simulink model "Final_Model_Building_2_AirflowAdded_BufferMode"  (R2022a)
settings: Solver=FixedStepAuto  StartTime=0.0  StopTime=24*3600  FixedStep=5  RelTol=1e-3
values from neighbouring files (symbols this model uses):
  Aux_Threshold = 52    [Setup_Code_EWASP_VC.m]
  buildingAge = 2005    [Setup_Code_EWASP_VC.m]
  ceilingHeight = 2.4    [Setup_Code_EWASP_VC.m]
  conductiveHconnectMatrix = [ ... (first row only)    [Setup_Code_EWASP_VC.m]
  cRoofGreen = 100000    [Setup_Code_EWASP_VC.m]
  Defrost_After_Time = 30    [Setup_Code_EWASP_VC.m]
  DHWDemandProfile = occFreegainHotwaterElecTestPassiveOcc3(:,3)    [Setup_Code_EWASP_VC.m]
  Elec_Max = Elec_Max*(30/24.2)    [Setup_Code_EWASP_VC.m]
  Elec_Mid = Elec_Mid*(30/24.2)    [Setup_Code_EWASP_VC.m]
  Elec_Min = Elec_Min*(30/24.2)    [Setup_Code_EWASP_VC.m]
  ElecDemandProfile = occFreegainHotwaterElecTestPassiveOcc3(:,4)    [Setup_Code_EWASP_VC.m]
  ElecFixed = [Elec_Max(6,2) Elec_Max(6,4) Elec_Max(6,6) Elec_Max(6,7) ... (first row only)    [Setup_Code_EWASP_VC.m]
  floorOrCeilingArea = floorOrCeilingArea*1.15    [Setup_Code_EWASP_VC.m]
  freegain = occFreegainHotwaterElecTestPassiveOcc3(:,2)-max(occupancy)*25    [Setup_Code_EWASP_VC.m]
  furnitureModelOn = 1    [Setup_Code_EWASP_VC.m]
  Heat_Max = Heat_Max*(30/24.2)    [Setup_Code_EWASP_VC.m]
  Heat_Mid = Heat_Mid*(30/24.2)    [Setup_Code_EWASP_VC.m]
  Heat_Min = Heat_Min*(30/24.2)    [Setup_Code_EWASP_VC.m]
  HeatFixed = [Heat_Max(6,2) Heat_Max(6,4) Heat_Max(6,6) Heat_Max(6,7) ... (first row only)    [Setup_Code_EWASP_VC.m]
  HeatingOnProfile = repmat(HeatingOnProfile,365,1)    [Setup_Code_EWASP_VC.m]
  HEX_ReturnLowerLimit = 52.5    [Setup_Code_EWASP_VC.m]
  HEX_ReturnUpperLimit = 55    [Setup_Code_EWASP_VC.m]
  LeakMultiplier = 1+(2*(rand()-0.5)/10)    [Setup_Code_EWASP_VC.m]
  maxOcc = max(occupancyProfile)    [Setup_Code_EWASP_VC.m]
  NESW_wallArea = max(NESW_Lengths*ceilingHeight-NESW_Windows,0)    [Setup_Code_EWASP_VC.m]
  NESW_Windows = [ ... (first row only)    [Setup_Code_EWASP_VC.m]
  numRooms = roomCount    [Setup_Code_EWASP_VC.m]
  occupancy = occupancyProfile    [Setup_Code_EWASP_VC.m]
  offsetDays = 0    [Setup_Code_EWASP_VC.m]
  overChargeSeries = repmat(overChargeSeries,365,1)    [Setup_Code_EWASP_VC.m]
  pumpChoice = pumpChoices(MinIndex,1)    [Setup_Code_EWASP_VC.m]
  pumpRamp = 180    [Setup_Code_EWASP_VC.m]
  RoofIrradiance = Flat_NS_EW_RoofIrradiance(:,1)    [Setup_Code_EWASP_VC.m]
  roofStartTemp = ones(11,1)*20    [Setup_Code_EWASP_VC.m]
  rooftype = 0    [Setup_Code_EWASP_VC.m]
  RoomDataMatrix = [zeros(1,12);ones(1,12)*wallDensity;zeros(1,12);ones(1,12)*wallU;ones(1,12)*windowU;ones(1,12)*floorU;ones(1,12)*ceilingU;zeros(1,12);windowArea, 0;floorOrCeilingArea;zeros(1,12);floorOrCeilingArea*ceilingHeight]    [Setup_Code_EWASP_VC.m]
  roomVol = roomVol*1.15    [Setup_Code_EWASP_VC.m]
  slabStartTemp = (GroundTempTimeSeries(offsetDays*1440+1,1)+thermostatSetting)/2    [Setup_Code_EWASP_VC.m]
  SlackRequest = zeros(1440,1)    [Setup_Code_EWASP_VC.m]
  SolarThermalExists = 0    [Setup_Code_EWASP_VC.m]
  SourceFixed = HeatFixed-ElecFixed    [Setup_Code_EWASP_VC.m]
  StateSeries = StateSeriesGenerator(22,7,1)    [Setup_Code_EWASP_VC.m]
  Tank_Lower_Temp = 49.5    [Setup_Code_EWASP_VC.m]
  Tank_Upper_Temp = 52    [Setup_Code_EWASP_VC.m]
  Tank_Volume_m3 = 0.15    [Setup_Code_EWASP_VC.m]
  TankHeatHour = randi([1 5])-1    [Setup_Code_EWASP_VC.m]
  upDown = [0;0;0;0;1;1;1;1;1;1;1]    [Setup_Code_EWASP_VC.m]
  wallStartTempExt = thermostatSetting*(0.266+0.00215*outdoorStartTemp+0.018*wallU+0.00113*outdoorStartTemp*wallU+0.0068*wallU^2)    [Setup_Code_EWASP_VC.m]
undefined symbols (not defined in the file or in its folder): a, ceilingU, condUDMatrix, convUDMatrix, deltaPEXPANDED_E, deltaPEXPANDED_E2, deltaPEXPANDED_N, deltaPEXPANDED_N2, deltaPEXPANDED_S, deltaPEXPANDED_S2, deltaPEXPANDED_W, deltaPEXPANDED_W2, DesiredDHWTemp, DesiredFlowTempVsInOutDeltaTemp, DiffuseHorizontal, DiscIntNeverNeededParam, DNI, dwnAndConcrete, ExtractRates, GroundTempTimeSeries, HCM, HCM2, HCM_closed, HCM_closed2, intermediateU, IsTop, massFlowMatrix, mechEfficiency, neighbourMatrix, numericalRoomUse, RadiatorMatrix, room2roomflowmatrix_E, room2roomflowmatrix_E2, room2roomflowmatrix_N, room2roomflowmatrix_N2, room2roomflowmatrix_S, room2roomflowmatrix_S2, room2roomflowmatrix_W, room2roomflowmatrix_W2, StateAirInEXPANDED_E, StateAirInEXPANDED_E2, StateAirInEXPANDED_N, StateAirInEXPANDED_N2, StateAirInEXPANDED_S, StateAirInEXPANDED_S2, StateAirInEXPANDED_W, StateAirInEXPANDED_W2, StateAirOutEXPANDED_E, StateAirOutEXPANDED_E2, StateAirOutEXPANDED_N, StateAirOutEXPANDED_N2, StateAirOutEXPANDED_S, StateAirOutEXPANDED_S2, StateAirOutEXPANDED_W, StateAirOutEXPANDED_W2, tankExists, TemperatureSeries, ThermostatBand, ThermostatSetting, Tin1 ... (+10)
libraries: simulink x6, dspsigops x4, dspmtrx3 x4, powerlib_meascontrol x3, carnot x3, dspstat3 x2
(part 1 of 29)
settings Model: Creator=cpp14rcj  LastModifiedBy=cpp14rcj
settings SolverCC: AlgebraicLoopSolver=TrustRegion
settings DataIOCC: SaveFormat=Array  ReturnWorkspaceOutputs=off
settings DebuggingCC: UnconnectedInputMsg=warning  UnconnectedOutputMsg=warning  UnconnectedLineMsg=warning  SFMachineParentedDataDiag=warning  ArithmeticOperatorsInVariantConditions=warning
settings SFSimCC: CustomCodeUndefinedFunction=UseInterfaceOnly
settings ConfigComp: PSAutoStubLUT=on

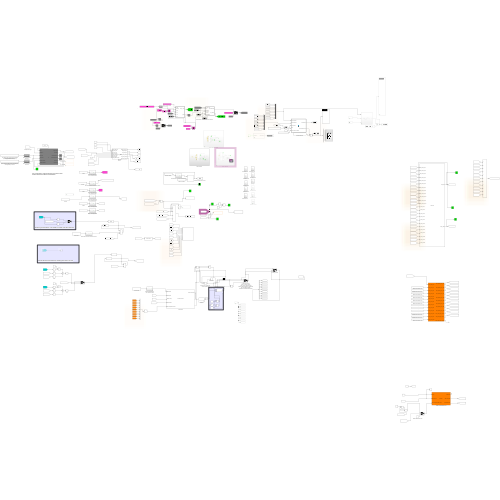
[thumbnail: Simulink's stored preview of the top-level diagram]
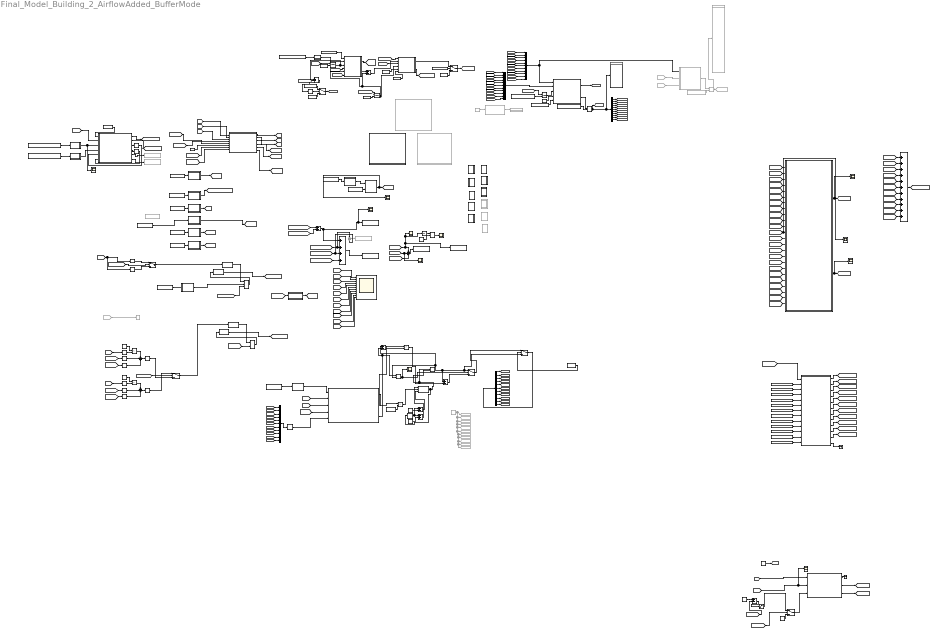
== system Final_Model_Building_2_AirflowAdded_BufferMode ==
  note: Prevents airflow from altering
      | extremely rapidly
  note: Handles logic that switches on the radiator circulation side of the buffer tank
  note: Grey Components: Components that are part of the model
      | White Components: Example Inputs/Outputs
  note: Handles the tank thermostat band, activating HP if buffer is too cool
  1 m : Relay  OnSwitchValue=12.1  OffSwitchValue=12  OnOutputValue=0  OffOutputValue=1  OutDataTypeStr=boolean
  1 m1 : Relay  Commented=on  OnSwitchValue=40  OffSwitchValue=37.5  OnOutputValue=0  OffOutputValue=1  OutDataTypeStr=boolean
  1 m10 : Relay  OnSwitchValue=7  OffSwitchValue=1  OutDataTypeStr=boolean
  1 m2 : Relay  OnSwitchValue=40  OffSwitchValue=37.5  OnOutputValue=0  OffOutputValue=1  OutDataTypeStr=boolean
  1 m3 : Relay  OnSwitchValue=40  OffSwitchValue=37.5  OnOutputValue=0  OffOutputValue=1  OutDataTypeStr=boolean
  1 m4 : Relay  OnSwitchValue=40  OffSwitchValue=37.5  OnOutputValue=0  OffOutputValue=1  OutDataTypeStr=boolean
  1 m5 : Relay  OnSwitchValue=3  OffSwitchValue=0.5  OutDataTypeStr=boolean
  1 m6 : Relay  OnSwitchValue=50  OffSwitchValue=47.5  OnOutputValue=0  OffOutputValue=1  OutDataTypeStr=boolean
  1 m7 : Relay  OnSwitchValue=50  OffSwitchValue=47.5  OnOutputValue=0  OffOutputValue=1  OutDataTypeStr=boolean
  1 m8 : Relay  OnSwitchValue=50  OffSwitchValue=47.5  OnOutputValue=0  OffOutputValue=1  OutDataTypeStr=boolean
  1 m9 : Relay  OnSwitchValue=3  OffSwitchValue=0.5  OutDataTypeStr=boolean
  ASHP_Subsystem : Subsystem
  ASHP_Subsystem_Variable : Subsystem  Commented=on
  Add : Sum  Inputs=11
  Add1 : Sum  Inputs=4
  Add2 : Sum
  Add3 : Sum  Inputs=+-
  Add4 : Sum
  Add5 : Sum  Inputs=+-
  Add6 : Sum  Inputs=+-
  Airflow Model : Subsystem
      mask Display:
      | disp('Air Flow Heat Loss')
      | port_label('input',1,'State Switch')
      | port_label('input',2,'Wind Speed')
      | port_label('input',3,'Outdoor Temp')
      | port_label('input',4,'Wind Direction')
      | port_label('input',5,'Room Temperature Vector')
      | port_label('output',1,'Room Loss Vector')
  Buffer Tank Model1 : Subsystem
      mask Display:
      | port_label('input', 1, 'Bottom_Node_dT')
      | port_label('input', 2, 'Mid_Node_dT')
      | port_label('input', 3, 'Top_Node_dT')
      | port_label('input', 4, 'HP_Flow_mdot')
      | port_label('input', 5, 'Central_Heating_Flow_mdot')
      | port_label('input', 6, 'Tank_Vol_litres')
      | port_label('input', 7, 'HP Flow Temp')
      | port_label('input', 8, 'Heating Return Temp')
      | 
      | port_label('output', 1, 'Bottom_Node_dT')
      | port_label('output', 2, 'Mid_Node_dT')
      | port_label('output', 3, 'Top_Node_dT')
      | port_label('output', 4, 'Bottom_Node_Temp')
      | port_label('output', 5, 'Top_Node_Temp')
      | port_label('output', 6, 'Mid_Node_Temp')
  "Bypass futher calcs, or ensure minimum loss is met by reducing heat gain in insert rooms - HAS NO EFFECT IF MECH VENTILATION IS NOT MODELLED, BUT THE MODEL IS MORE RELIABLE IN THIS INSTANCE ANYWAY" : Switch  Criteria=u2 > Threshold  Threshold=0.5  SaturateOnIntegerOverflow=off  InputSameDT=off
  CondLossIntermediate : Subsystem  Commented=on
      mask Display:
      | port_label('input',1, 'RoomNum')
      | port_label('output',1,'IntCondGain')
  Constant : Constant  Value=3600
  Constant1 : Constant  Commented=on  Value=0
  Constant10 : Constant  Value=300
  Constant11 : Constant  Value=maxOcc*0.054/2
  Constant12 : Constant  Value=2.1
  Constant13 : Constant  Value=20*ones(11,11)
  Constant14 : Constant  Value=0
  Constant15 : Constant  Value=conductiveHconnectMatrix
  Constant2 : Constant  Value=25
  Constant21 : Constant  Value=buildingAge
  Constant3 : Constant  Value=10
  Constant4 : Constant  Commented=on  Value=11
  Constant5 : Constant  Value=25
  Constant6 : Constant  Value=10
  Constant7 : Constant  Value=0
  Constant8 : Constant  Value=20
  Constant9 : Constant  Value=50
  Data Type Conversion{,1..3} (4 alike) : DataTypeConversion  OutDataTypeStr=double  SaturateOnIntegerOverflow=off  RndMeth=Floor
  Delay3 : Delay  DelayLength=1  InitialCondition=0
  Delay4 : Delay  DelayLength=1  InitialCondition=0
  Delay5 : Delay  DelayLength=1  InitialCondition=0
  Demux : Demux  Outputs=11
  Demux1 : Demux  Outputs=11
  Digital Clock3 : DigitalClock  SampleTime=5
  Discrete-Time Integrator : DiscreteIntegrator  InitialConditionSource=external  InitialCondition=20  SampleTime=-1  ICPrevOutput=DiscIntNeverNeededParam  ICPrevScaledInput=DiscIntNeverNeededParam
  Discrete-Time Integrator1 : DiscreteIntegrator  InitialConditionSource=external  SampleTime=-1  ICPrevOutput=DiscIntNeverNeededParam  ICPrevScaledInput=DiscIntNeverNeededParam
  Display1 : Display
  Display2 : Display  Commented=on
  Display3 : Display  Commented=on
  Divide : Product  Inputs=*/
  From11 : From
  From14 : From  Commented=on  GotoTag=T_Buffer
  From63 : From  Commented=on  GotoTag=windSpeed  TagVisibility=global
  From87 : From  Commented=on  GotoTag=T_Out  TagVisibility=global
  GSHP_Subsystem : Subsystem  Commented=on
  Goto11 : Goto  Commented=on  GotoTag=AirLoss5  TagVisibility=global
  Goto12 : Goto  Commented=on  GotoTag=AirLoss6  TagVisibility=global
  Goto16 : Goto  Commented=on  GotoTag=AirLoss7  TagVisibility=global
  Goto17 : Goto
  Goto18 : Goto  Commented=on  GotoTag=AirLoss8  TagVisibility=global
  Goto19 : Goto  Commented=on  GotoTag=AirLoss9  TagVisibility=global
  Goto20 : Goto  Commented=on  GotoTag=AirLoss10  TagVisibility=global
  Goto21 : Goto  Commented=on  GotoTag=AirLoss11  TagVisibility=global
  Goto33 : Goto  Commented=on  GotoTag=deltaTRoofNodes  TagVisibility=global
  Goto5 : Goto  Commented=on  GotoTag=AirLoss1  TagVisibility=global
  Goto7 : Goto  Commented=on  GotoTag=AirLoss2  TagVisibility=global
  Goto8 : Goto  Commented=on  GotoTag=AirLoss3  TagVisibility=global
  Goto9 : Goto  Commented=on  GotoTag=AirLoss4  TagVisibility=global
  Heat sys act?1 : Constant  Value=HeatingOnProfile
  Heat sys act?2 : Constant  Value=StateSeries
  If predicted loss exceeds (is more negative than) minimum possible loss : RelationalOperator  OutDataTypeStr=boolean  RndMeth=Simplest  InputSameDT=off
  Integrator : Integrator
  Logical Operator1 : Logic  AllPortsSameDT=off  OutDataTypeStr=boolean
  Logical Operator5 : Logic  Inputs=3  AllPortsSameDT=off  OutDataTypeStr=boolean
  MATLAB Function : MATLAB Function  TreatAsAtomicUnit=on
  MATLAB Function1 : MATLAB Function  TreatAsAtomicUnit=on
  MATLAB Function2 : MATLAB Function  TreatAsAtomicUnit=on
  MATLAB Function3 : MATLAB Function  TreatAsAtomicUnit=on
  Massflow when system is off3 : Constant  Value=0
  Massflow when system is on1 : Constant  Value=massFlowMatrix(1,3)
  Massflow when system is on10 : Constant  Value=massFlowMatrix(1,11)
  Massflow when system is on11 : Constant  Value=massFlowMatrix(1,10)
  Massflow when system is on13 : Constant  Value=massFlowMatrix(1,2)
  Massflow when system is on2 : Constant  Value=massFlowMatrix(1,1)
  Massflow when system is on3 : Constant  Value=massFlowMatrix(1,6)
  Massflow when system is on4 : Constant  Value=massFlowMatrix(1,5)
  Massflow when system is on5 : Constant  Value=massFlowMatrix(1,9)
  Massflow when system is on6 : Constant  Value=massFlowMatrix(1,8)
  Massflow when system is on7 : Constant  Value=massFlowMatrix(1,4)
  Massflow when system is on8 : Constant  Value=massFlowMatrix(1,7)
  Massflow when system is on9 : Constant  Value=massFlowMatrix(1,12)
  Minus : Sum  Inputs=+-
  Mux : Mux  Inputs=11
  Mux1 : Mux  Inputs=11
  Offset Independent time series element selector : Subsystem
  Offset Independent time series element selector1 : Subsystem
  Offset Independent time series element selector2 : Subsystem
  Plus : Sum  Inputs=+-
  Plus1 : Sum  Inputs=+-
  Predicted loss1 : Scope
  Product : Product  Inputs=*/
  Product{1..4} (4 alike) : Product
  Product5 : Product  Inputs=*/
  Product6 : Product  Commented=on  Inputs=*/
  Radiator w/Thermostatic Control : Subsystem  mask{DeltaT_Nominal=40, Power_Nominal=100, TRV_Therm_Setpoint=1000, Water_Volume=4}
      mask prompts: DeltaT_Nominal "DeltaT_Nominal (oC)"; Power_Nominal "Power_Nominal (W)"; TRV_Therm_Setpoint "TRV/Thermostat Setpoint (oC)"; Water_Volume "Water Volume (l)"
      mask Display:
      | disp('Radiator')
      | port_label('input', 1, 'Troom')
      | port_label('input', 2, 'Water Temp In')
      | port_label('input', 3, 'Water Mass Flow Rate (open)')
      | port_label('output', 1, 'Qdot2room')
      | port_label('output', 2, 'Water Temp Out')
      | port_label('output', 3, 'Actual Mass Flow')
      | %image('C:\Users\cpp14rcj\Desktop\MODEL IMAGES\radiator-67-778961.png')
  Relay1 : Relay  OnSwitchValue=ThermostatSetting  OffSwitchValue=ThermostatSetting-ThermostatBand  OnOutputValue=0  OffOutputValue=1  OutDataTypeStr=boolean
  Saturation Dynamic : simulink/Discontinuities/Saturation Dynamic  OutMin=[]  OutMax=[]  OutDataTypeStr=Inherit: Same as second input  OutDataType=fixdt(1, 16)  OutScaling=2^-10  DoSatur=off
  Saturation1 : Saturate  UpperLimit=1000  LowerLimit=0
  Scope{,1..3,6,10..12,19,27} (10 alike) : Scope
  Scope5 : Scope  NumInputPorts=11
  Select Correct Element from Array1 : Subsystem
  Select Correct Element from Array2 : Subsystem
  "Select correct element from array, considering offset" : Subsystem
  "Select correct element from array, considering offset1" : Subsystem
  "Select correct element from array, considering offset2" : Subsystem
  "Select correct element from array, considering offset3" : Subsystem
  "Select correct element from array, considering offset4" : Subsystem
  "Select correct element from array, considering offset5" : Subsystem
  Selector2 : Selector  NumberOfDimensions=2  InputPortWidth=3  IndexOptions=Index vector (dialog),Index vector (dialog)  Indices=1:11,1  OutputSizes=1,1
  Subsystem : Subsystem
      mask Display:
      | disp('Flow mixer')
      | port_label('input', 13, 'T_return_rad1')
      | port_label('input', 14, 'T_return_rad2')
      | port_label('input', 15, 'T_return_rad3')
      | port_label('input', 16, 'T_return_rad4')
      | port_label('input', 17, 'T_return_rad5')
      | port_label('input', 18, 'T_return_rad6')
      | port_label('input', 19, 'T_return_rad7')
      | port_label('input', 20, 'T_return_rad8')
      | port_label('input', 21, 'T_return_rad9')
      | port_label('input', 22,'T_return_rad10')
      | port_label('input', 23,'T_return_rad11')
      | port_label('input', 24,'T_return_rad12')
      | 
      | port_label('input', 1, 'mdot_return_rad1')
      | port_label('input', 2, 'mdot_return_rad2')
      | port_label('input', 3, 'mdot_return_rad3')
      | port_label('input', 4, 'mdot_return_rad4')
      | port_label('input', 5, 'mdot_return_rad5')
      | port_label('input', 6, 'mdot_return_rad6')
      | port_label('input', 7, 'mdot_return_rad7')
      | port_label('input', 8, 'mdot_return_rad8')
      | port_label('input', 9, 'mdot_return_rad9')
      | port_label('input', 10, 'mdot_return_rad10')
      | port_label('input', 11, 'mdot_return_rad11')
      | port_label('input', 12, 'mdot_return_rad12')
      | 
      | port_label('output', 1, 'mdot_total')
      | port_label('output', 2, 'Temp_mixed')
  Subsystem1 : Subsystem
      mask Display:
      | port_label('input', 1, 'mdot_return_rad1')
      | port_label('input', 2, 'mdot_open_rad1')
      | port_label('input', 3, 'mdot_open_rad2')
      | port_label('input', 4, 'mdot_open_rad3')
      | port_label('input', 5, 'mdot_open_rad4')
      | port_label('input', 6, 'mdot_open_rad5')
      | port_label('input', 7, 'mdot_open_rad6')
      | port_label('input', 8, 'mdot_open_rad7')
      | port_label('input', 9, 'mdot_open_rad8')
      | port_label('input', 10, 'mdot_open_rad9')
      | port_label('input', 11, 'mdot_open_rad10')
      | port_label('input', 12, 'mdot_open_rad11')
      | port_label('input', 13, 'mdot_open_rad12')
      | 
      | 
      | port_label('output', 1, 'mdot_actual_open_rad1')
      | port_label('output', 2, 'mdot_actual_open_rad2')
      | port_label('output', 3, 'mdot_actual_open_rad3')
      | port_label('output', 4, 'mdot_actual_open_rad4')
      | port_label('output', 5, 'mdot_actual_open_rad5')
      | port_label('output', 6, 'mdot_actual_open_rad6')
      | port_label('output', 7, 'mdot_actual_open_rad7')
      | port_label('output', 8, 'mdot_actual_open_rad8')
      | port_label('output', 9, 'mdot_actual_open_rad9')
      | port_label('output', 10, 'mdot_actual_open_rad10')
      | port_label('output', 11, 'mdot_actual_open_rad11')
      | port_label('output', 12, 'mdot_actual_open_rad12')
  Subsystem2 : Subsystem
      mask Display: disp('10 min Limiter')
  Subsystem3 : Subsystem
  Subsystem4 : Subsystem  Commented=on
  Subsystem_Room1 : Subsystem
  Subsystem_Room10 : Subsystem  Commented=on
  Subsystem_Room11 : Subsystem  Commented=on
  Subsystem_Room2 : Subsystem
  Subsystem_Room3 : Subsystem
  Subsystem_Room4 : Subsystem
  Subsystem_Room5 : Subsystem
  Subsystem_Room6 : Subsystem
  Subsystem_Room7 : Subsystem
  Subsystem_Room8 : Subsystem
  Subsystem_Room9 : Subsystem  Commented=on
  Sum : Sum  Inputs=3
  Sum of Elements1 : Sum  Inputs=+
  Sum1 : Sum  Inputs=3
  Sum5 : Sum  Inputs=+++
  Sum6 : Sum  Commented=on
  Switch{,1..3,7} (5 alike) : Switch  Criteria=u2 > Threshold  Threshold=0.5  SaturateOnIntegerOverflow=off  InputSameDT=off
  Temp Hex : DiscreteIntegrator  InitialConditionSource=external  InitialCondition=20  SampleTime=-1  ICPrevOutput=DiscIntNeverNeededParam  ICPrevScaledInput=DiscIntNeverNeededParam
  Terminator1 : Terminator
  Terminator13 : Terminator
  Tinitial10 : Constant  Value=0.2
  Tinitial16 : Constant  Value=20
  Tinitial18 : Constant  Value=LeakMultiplier
  To Workspace : ToWorkspace  VariableName=CalculatedProfile  SaveFormat=Timeseries  SampleTime=-1
  To Workspace1 : ToWorkspace  VariableName=CalculatedHeatOutProfile  SaveFormat=Timeseries  SampleTime=-1
  To Workspace2 : ToWorkspace  Commented=on  VariableName=DHWonly  SaveFormat=Timeseries  SampleTime=-1
  To Workspace3 : ToWorkspace  Commented=on  VariableName=MO1  SaveFormat=Timeseries  SampleTime=-1
  To Workspace4 : ToWorkspace  Commented=on  VariableName=MO2  SaveFormat=Timeseries  SampleTime=-1
  To Workspace5 : ToWorkspace  VariableName=ElecSHonly  SaveFormat=Timeseries  SampleTime=-1
  To Workspace6 : ToWorkspace  VariableName=SHonly  SaveFormat=Timeseries  SampleTime=-1
  Vector Concatenate : Concatenate  NumInputs=11
  angle that DNI hits a NEWS wall/window as a function of time1 : Constant  Value=RoofIrradiance
  angle that DNI hits a NEWS wall/window as a function of time2 : Constant  Value=SolarThermalExists
  assign 1m2 per occupant : Constant  Value=maxOcc
  coil watermass - roughly 8m coil with 9mm diameter : Constant  Value=0.55
  effective coil HEX u value : Constant  Value=11
  on? (I/O)1 : Constant  Value=GroundTempTimeSeries  OutDataTypeStr=double
  on? (I/O)2 : Constant  Commented=on  Value=TemperatureSeries  OutDataTypeStr=double
  on? (I/O)3 : Constant  Value=windSpeedSeries  OutDataTypeStr=double
  on? (I/O)4 : Constant  Value=WDS_Numerical  OutDataTypeStr=double
  on? (I/O)5 : Constant  Value=ElecDemandProfile  OutDataTypeStr=double
  on? (I/O)6 : Constant  Value=overChargeSeries  OutDataTypeStr=double
  on? (I/O)7 : Constant  Value=-5  OutDataTypeStr=double
  only allows supressor if building is passive : Switch  Threshold=2020  SaturateOnIntegerOverflow=off  InputSameDT=off
  roomAirHeatCapcities : Constant  Value=1000*1.225*roomVol(1,1:11)'
  roomAirHeatCapcities1 : Constant  Commented=on  Value=1000*1.225*roomVol(1,1:11)'
  "vector Representing request to charge a 2kWh (7.2 MJ) (vector results in charging between 00:00 and 03:00, and brings battery to 75% SoC" : Constant  Value=[zeros(1440,1)]
  vector Representing request to slacken deadband at any given minute of the day (sends request between 18:00 and 21:00) : Constant  Value=SlackRequest
  watts per occupant : Constant  Value=freegain  OutDataTypeStr=double
  watts per occupant1 : Constant  Value=numRooms  OutDataTypeStr=double
  tag scope: AirLoss10=global, AirLoss11=global, AirLoss1=global, AirLoss2=global, AirLoss3=global, AirLoss4=global, AirLoss5=global, AirLoss6=global, AirLoss7=global, AirLoss8=global, AirLoss9=global, Allowed_on=global, Global_Control_Signal=global, Ground=global, MassFlowTotal=global, MassFlow_Full_Open_10=global, MassFlow_Full_Open_11=global, MassFlow_Full_Open_1=global, MassFlow_Full_Open_2=global, MassFlow_Full_Open_3=global, MassFlow_Full_Open_4=global, MassFlow_Full_Open_5=global, MassFlow_Full_Open_6=global, MassFlow_Full_Open_7=global, MassFlow_Full_Open_8=global, MassFlow_Full_Open_9=global, Mdot_Actual_12=global, MixedTemp=global, Occ_Free_Gain=global, OverCharge=global, Pump_Return=global, RAD_TOTAL=global, SolarHeatToWater=global, THB_In=global, T_12=global, T_Out=global, T_return_R12=global, deltaTPartition10=global, deltaTPartition11=global, deltaTPartition1=global, deltaTPartition2=global, deltaTPartition3=global, deltaTPartition4=global, deltaTPartition5=global, deltaTPartition6=global, deltaTPartition7=global, deltaTPartition8=global, deltaTPartition9=global, pump_control_signal=global, windDirection=global, windSpeed=global
  wires:
  Data Type Conversion2/1 -> Logical Operator5/1
  Logical Operator5/1 -> Data Type Conversion/1
  Subsystem/2(Out2) -> Scope12/1, [MixedTemp]
  [T_return_R12] -> Subsystem/24(In24)
  [T_return_R11] -> Subsystem/23(In23)
  [T_return_R6] -> Subsystem/18(In18)
  [T_return_R7] -> Subsystem/19(In19)
  [T_return_R8] -> Subsystem/20(In20)
  [T_return_R9] -> Subsystem/21(In21)
  [T_return_R4] -> Subsystem/16(In16)
  [T_return_R1] -> Subsystem/13(In13)
  [Mdot_Actual_11] -> Subsystem/11(In11)
  [Mdot_Actual_12] -> Scope19/1, Subsystem/12(In12)
  [Mdot_Actual_8] -> Subsystem/8(In8)
  [T_return_R5] -> Subsystem/17(In17)
  [Mdot_Actual_5] -> Subsystem/5(In5)
  [Mdot_Actual_6] -> Subsystem/6(In6)
  [Mdot_Actual_4] -> Subsystem/4(In4)
  [Mdot_Actual_10] -> Subsystem/10(In10)
  [Mdot_Actual_3] -> Subsystem/3(In3)
  [Mdot_Actual_2] -> Subsystem/2(In2)
  [T_return_R10] -> Subsystem/22(In22)
  [Mdot_Actual_9] -> Subsystem/9(In9)
  [Mdot_Actual_1] -> Subsystem/1(In1)
  [T_return_R3] -> Subsystem/15(In15)
  [Mdot_Actual_7] -> Subsystem/7(In7)
  [T_return_R2] -> Subsystem/14(In14)
  [pump_control_signal] -> Subsystem1/1(In1)
  Massflow when system is on2/1 -> Subsystem1/2(In2)
  Massflow when system is on13/1 -> Subsystem1/3(In3)
  Massflow when system is on1/1 -> Subsystem1/4(In4)
  Subsystem1/1(Out1) -> [MassFlow_Full_Open_1]
  Subsystem1/2(Out2) -> [MassFlow_Full_Open_2]
  Subsystem1/3(Out3) -> [MassFlow_Full_Open_3]
  Subsystem1/4(Out4) -> [MassFlow_Full_Open_4]
  Subsystem1/5(Out5) -> [MassFlow_Full_Open_5]
  Subsystem1/6(Out6) -> [MassFlow_Full_Open_6]
  Subsystem1/7(Out7) -> [MassFlow_Full_Open_7]
  Subsystem1/8(Out8) -> [MassFlow_Full_Open_8]
  Subsystem1/9(Out9) -> [MassFlow_Full_Open_9]
  Subsystem1/11(Out11) -> [MassFlow_Full_Open_11]
  Subsystem1/12(Out12) -> Terminator13/1
  Data Type Conversion/1 -> [pump_control_signal]
  Subsystem/1(Out1) -> Scope10/1, [MassFlowTotal]
  [T_4] -> Scope5/4
  [T_5] -> Scope5/5
  [T_6] -> Scope5/6
  [T_1] -> Scope5/1
  [T_2] -> Scope5/2
  [T_3] -> Scope5/3
  [T_7] -> Scope5/7
  [T_8] -> Scope5/8
  [T_9] -> Scope5/9
  [T_10] -> Scope5/10
  [T_11] -> Scope5/11
  [hysteresis] -> Subsystem2/1(In1)
  Subsystem2/1(Out1) -> [Allowed_on]
  Tinitial16/1 -> [T_12]
  [T_12] -> Radiator w/Thermostatic Control/1(In1)
  [THB_In] -> Scope/1, Radiator w/Thermostatic Control/2(In2)
  Tinitial10/1 -> Minus/1
  Minus/1 -> Saturation1/1
  [RAD_TOTAL] -> Minus/2
  Saturation1/1 -> Switch7/1
  Radiator w/Thermostatic Control/2(Out2) -> [T_return_R12]
  Radiator w/Thermostatic Control/3(Out3) -> [Mdot_Actual_12]
  Subsystem1/10(Out10) -> [MassFlow_Full_Open_10]
  Add/1 -> [RAD_TOTAL]
  Massflow when system is off3/1 -> Switch7/3
  [pump_control_signal] -> Switch7/2
  Switch7/1 -> Radiator w/Thermostatic Control/3(In3)
  [Mdot_Actual_2] -> Add/2
  [Mdot_Actual_4] -> Add/4
  [Mdot_Actual_7] -> Add/7
  [Mdot_Actual_9] -> Add/9
  [Mdot_Actual_11] -> Add/11
  [Mdot_Actual_6] -> Add/6
  [Mdot_Actual_8] -> Add/8
  [Mdot_Actual_10] -> Add/10
  [Mdot_Actual_1] -> Add/1
  [Mdot_Actual_3] -> Add/3
  [Mdot_Actual_5] -> Add/5
  Constant4/1 -> CondLossIntermediate/1(In1)
  CondLossIntermediate/1(Out1) -> Display3/1
  [windDirection] -> Airflow Model/4(In4)
  Vector Concatenate/1 -> Selector2/1
  Heat sys act?2/1 -> "Select correct element from array, considering offset4"/1(In1)
  [T_Out] -> Airflow Model/3(In3)
  Demux/1 -> [AirLoss1]
  Demux/2 -> [AirLoss2]
  Demux/3 -> [AirLoss3]
  Demux/4 -> [AirLoss4]
  Demux/5 -> [AirLoss5]
  Demux/6 -> [AirLoss6]
  Demux/7 -> [AirLoss7]
  Demux/8 -> [AirLoss8]
  Demux/9 -> [AirLoss9]
  Demux/10 -> [AirLoss10]
  Demux/11 -> [AirLoss11]
  [T_1] -> Vector Concatenate/1
  [T_2] -> Vector Concatenate/2
  [T_3] -> Vector Concatenate/3
  [T_4] -> Vector Concatenate/4
  [T_5] -> Vector Concatenate/5
  [T_6] -> Vector Concatenate/6
  [T_7] -> Vector Concatenate/7
  [T_8] -> Vector Concatenate/8
  [T_9] -> Vector Concatenate/9
  [T_10] -> Vector Concatenate/10
  [T_11] -> Vector Concatenate/11
  Selector2/1 -> Airflow Model/5(In5)
  "Select correct element from array, considering offset4"/1(Out1) -> Airflow Model/1(In1)
  on? (I/O)1/1 -> "Select correct element from array, considering offset"/1(In1)
  on? (I/O)3/1 -> "Select correct element from array, considering offset2"/1(In1)
  "Select correct element from array, considering offset3"/1(Out1) -> [windDirection]
  on? (I/O)4/1 -> "Select correct element from array, considering offset3"/1(In1)
  "Select correct element from array, considering offset"/1(Out1) -> [Ground]
  [windSpeed] -> Airflow Model/2(In2)
  Radiator w/Thermostatic Control/1(Out1) -> Terminator1/1
  on? (I/O)5/1 -> Offset Independent time series element selector/1(In1)
  Offset Independent time series element selector/1(Out1) -> [ApplianceAndLightElectricalPower]
  Offset Independent time series element selector1/1(Out1) -> Logical Operator5/2
  Heat sys act?1/1 -> Offset Independent time series element selector1/1(In1)
  Product2/1 -> Saturation Dynamic/2
  Tinitial18/1 -> Product2/2
  [ElectrifiedHeatToWater] -> Sum6/1, Add1/2
  Add1/1 -> To Workspace/1
  Airflow Model/1(Out1) -> Product2/1
  Massflow when system is on3/1 -> Subsystem1/7(In7)
  Massflow when system is on4/1 -> Subsystem1/6(In6)
  Massflow when system is on7/1 -> Subsystem1/5(In5)
  Massflow when system is on11/1 -> Subsystem1/11(In11)
  Massflow when system is on9/1 -> Subsystem1/13(In13)
  Massflow when system is on10/1 -> Subsystem1/12(In12)
  Massflow when system is on5/1 -> Subsystem1/10(In10)
  Massflow when system is on6/1 -> Subsystem1/9(In9)
  Massflow when system is on8/1 -> Subsystem1/8(In8)
  Sum5/1 -> To Workspace1/1
  [HeatToWater] -> Scope27/1, Sum5/2
  [AuxHeatToWater] -> Sum5/3
  Sum6/1 -> To Workspace2/1
  [AuxHeatToWater] -> Sum6/2, Add1/3
  on? (I/O)7/1 -> "Select correct element from array, considering offset1"/1(In1)
  Delay4/1 -> MATLAB Function/6(ModelFeedbackIn2)
  Digital Clock3/1 -> MATLAB Function/1(clock)
  vector Representing request to slacken deadband at any given minute of the day (sends request between 18:00 and 21:00)/1 -> Select Correct Element from Array1/1(In1)
  "vector Representing request to charge a 2kWh (7.2 MJ) (vector results in charging between 00:00 and 03:00, and brings battery to 75% SoC"/1 -> Select Correct Element from Array2/1(In1)
  Delay3/1 -> MATLAB Function/5(ModelFeedbackIn)
  MATLAB Function/4(ModelFeedbackOut2) -> Delay4/1
  MATLAB Function/6(MonitorOut2) -> To Workspace4/1
  MATLAB Function/2(RelaxBand) -> [RelaxBand]
  Select Correct Element from Array2/1(Out1) -> MATLAB Function/4(ExternalIn2)
  Select Correct Element from Array1/1(Out1) -> Scope11/1, MATLAB Function/3(ExternalIn)
  MATLAB Function/5(MonitorOut) -> To Workspace3/1
  MATLAB Function/3(ModelFeedbackOut) -> Delay3/1
  [T_5] -> MATLAB Function/2(HeatSysIn)
  Switch/1 -> Data Type Conversion2/1
  Relay1/1 -> Switch/3
  [T_1] -> Relay1/1, 1 m/1
  1 m/1 -> Switch/1
  [RelaxBand] -> Switch/2
  Constant1/1 -> Goto21/1, Goto20/1, Goto19/1, Goto18/1, Goto16/1, Goto12/1, Goto11/1, Goto9/1, Goto8/1, Goto7/1, Goto5/1
  Saturation Dynamic/1 -> Delay5/1, Add5/1, only allows supressor if building is passive/3, "Bypass futher calcs, or ensure minimum loss is met by reducing heat gain in insert rooms - HAS NO EFFECT IF MECH VENTILATION IS NOT MODELLED, BUT THE MODEL IS MORE RELIABLE IN THIS INSTANCE ANYWAY"/1, Sum of Elements1/1
  Delay5/1 -> Add3/1, Add2/1
  Constant2/1 -> Add3/2
  Constant5/1 -> Add2/2
  Add3/1 -> Saturation Dynamic/3
  Add2/1 -> Saturation Dynamic/1
  "Select correct element from array, considering offset1"/1(Out1) -> [T_Out]
  MATLAB Function/1(SystemActive) -> [SystemActiveInterractor]
  Add4/1 -> Add1/1, Scope3/1, To Workspace5/1
  Integrator/1 -> Divide/1
  Divide/1 -> Scope2/1
  Constant/1 -> Divide/2
  [ElectrifiedHeatToSpaceG] -> Add4/1
  [ElectrifiedHeatToSpace] -> Add4/2
  watts per occupant1/1 -> Product/2
  Product/1 -> Scope6/1, [Occ_Free_Gain]
  watts per occupant/1 -> Offset Independent time series element selector2/1(In1)
  Offset Independent time series element selector2/1(Out1) -> Product/1
  [HeatToSpace] -> To Workspace6/1, Integrator/1, Scope1/1, Sum5/1
  [ApplianceAndLightElectricalPower] -> Add1/4
  Airflow Model/2(TempFixForMechSystems) -> Product1/1
  Airflow Model/3(MinimumAirlossPhysicallyPossible) -> If predicted loss exceeds (is more negative than) minimum possible loss/1, Add6/2
  Sum of Elements1/1 -> If predicted loss exceeds (is more negative than) minimum possible loss/2, Add6/1
  If predicted loss exceeds (is more negative than) minimum possible loss/1 -> Predicted loss1/1, "Bypass futher calcs, or ensure minimum loss is met by reducing heat gain in insert rooms - HAS NO EFFECT IF MECH VENTILATION IS NOT MODELLED, BUT THE MODEL IS MORE RELIABLE IN THIS INSTANCE ANYWAY"/2
  only allows supressor if building is passive/1 -> Demux/1
  Add6/1 -> Product1/2
  Product1/1 -> Add5/2
  Add5/1 -> "Bypass futher calcs, or ensure minimum loss is met by reducing heat gain in insert rooms - HAS NO EFFECT IF MECH VENTILATION IS NOT MODELLED, BUT THE MODEL IS MORE RELIABLE IN THIS INSTANCE ANYWAY"/3
  "Bypass futher calcs, or ensure minimum loss is met by reducing heat gain in insert rooms - HAS NO EFFECT IF MECH VENTILATION IS NOT MODELLED, BUT THE MODEL IS MORE RELIABLE IN THIS INSTANCE ANYWAY"/1 -> only allows supressor if building is passive/1
  Constant21/1 -> only allows supressor if building is passive/2
  "Select correct element from array, considering offset2"/1(Out1) -> [windSpeed]
  From11/1 -> Buffer Tank Model1/1(In1)
  [C] -> Buffer Tank Model1/3(In3)
  Buffer Tank Model1/3(Out3) -> [C]
  Constant10/1 -> Buffer Tank Model1/6(In6)
  [HeatPumpFlow] -> Buffer Tank Model1/5(In5)
  [B] -> Buffer Tank Model1/2(In2)
  Buffer Tank Model1/2(Out2) -> [B]
  Buffer Tank Model1/1(Out1) -> Goto17/1
  [MassFlowTotal] -> Buffer Tank Model1/4(In4)
  [THB_In_Pre] -> Buffer Tank Model1/7(In7)
  [MixedTemp] -> Buffer Tank Model1/8(In8)
  Buffer Tank Model1/5(Out5) -> [THB_In]
  Buffer Tank Model1/4(Out4) -> [Pump_Return]
  Buffer Tank Model1/6(Out6) -> [T_Buffer]
  Data Type Conversion3/1 -> Logical Operator1/1
  From14/1 -> 1 m1/1
  Logical Operator1/1 -> Data Type Conversion1/1
  Data Type Conversion1/1 -> [Global_Control_Signal]
  [Allowed_on] -> Logical Operator1/2
  [SystemActiveInterractor] -> Logical Operator5/3
  [T_Buffer] -> 1 m2/1
  [THB_In] -> 1 m3/1
  [Pump_Return] -> 1 m4/1
  1 m2/1 -> Product3/2
  Constant3/1 -> Product3/1
  Product3/1 -> Sum/1
  1 m3/1 -> Sum/2
  1 m4/1 -> Sum/3
  Sum/1 -> 1 m5/1
  Constant6/1 -> Product4/1
  1 m7/1 -> Sum1/2
  [THB_In] -> 1 m7/1
  1 m6/1 -> Product4/2
  Product4/1 -> Sum1/1
  Sum1/1 -> 1 m9/1
  [Pump_Return] -> 1 m8/1
  [T_Buffer] -> 1 m6/1
  1 m8/1 -> Sum1/3
  1 m9/1 -> Switch1/1
  1 m5/1 -> Switch1/3
  Switch1/1 -> Data Type Conversion3/1
  [OverCharge] -> Switch1/2
  on? (I/O)6/1 -> "Select correct element from array, considering offset5"/1(In1)
  "Select correct element from array, considering offset5"/1(Out1) -> [OverCharge]
  assign 1m2 per occupant/1 -> MATLAB Function1/1(A_COLL)
  [dT_Panel] -> Discrete-Time Integrator/1
  Discrete-Time Integrator/1 -> MATLAB Function1/3(T_panel), Plus1/1
  MATLAB Function1/1(delta_T_Panel) -> [dT_Panel]
  [T_Out] -> MATLAB Function1/4(T_amb)
  Constant8/1 -> Discrete-Time Integrator/2
  1 m10/1 -> Switch2/2
  [tank_bottom_temp] -> Plus1/2
  Plus1/1 -> 1 m10/1
  Constant11/1 -> Switch2/1
  Constant14/1 -> Switch2/3
  MATLAB Function1/2(T_outlet) -> Plus/1
  Switch2/1 -> [mDotPanel]
  Temp Hex/1 -> MATLAB Function2/4(Hex_Temp), MATLAB Function1/5(T_inlet), Plus/2
  Constant9/1 -> Temp Hex/2
  effective coil HEX u value/1 -> MATLAB Function2/5(Hex_Uval)
  [dT_HEXsolar] -> Temp Hex/1
  Plus/1 -> MATLAB Function2/2(T_diff)
  coil watermass - roughly 8m coil with 9mm diameter/1 -> MATLAB Function2/6(coilWaterMass)
  MATLAB Function2/1(solarHeatToWater) -> Switch3/1
  [tank_bottom_temp] -> MATLAB Function2/1(T_bottom_Tank)
  [mDotPanel] -> MATLAB Function2/3(mDotPanel)
  [mDotPanel] -> MATLAB Function1/6(m_dot)
  angle that DNI hits a NEWS wall/window as a function of time1/1 -> Subsystem3/1(In1)
  Subsystem3/1(Out1) -> MATLAB Function1/2(Q_SOLAR)
  MATLAB Function2/2(dT_HEXsolar) -> [dT_HEXsolar]
  Switch3/1 -> [SolarHeatToWater]
  Constant7/1 -> Switch3/3
  angle that DNI hits a NEWS wall/window as a function of time2/1 -> Switch3/2
  [Q_rad_win3] -> Mux1/3
  [T_5] -> Mux/5
  Product5/1 -> [deltaTRoom], Display1/1, Demux1/1
  [T_2] -> Mux/2
  Demux1/1 -> [deltaTPartition1]
  Mux/1 -> Subsystem4/1(In1), MATLAB Function3/1(RoomTempVector)
  roomAirHeatCapcities1/1 -> Product6/2
  MATLAB Function3/1(SurfaceDeltaT) -> [deltaTWalls]
  [Q_rad_win6] -> Mux1/6
  Demux1/5 -> [deltaTPartition5]
  Demux1/2 -> [deltaTPartition2]
  [Q_rad_win8] -> Mux1/8
  [T_8] -> Mux/8
  [Q_rad_win2] -> Mux1/2
  [Q_rad_win7] -> Mux1/7
  Demux1/7 -> [deltaTPartition7]
  [Q_rad_win10] -> Mux1/10
  [Q_rad_win9] -> Mux1/9
  Constant12/1 -> MATLAB Function3/4(wallU)
  MATLAB Function3/2(RoomHeatLossVector) -> Product5/1
  Constant15/1 -> MATLAB Function3/5(conductiveHconnectMatrix)
  [T_4] -> Mux/4
  Demux1/8 -> [deltaTPartition8]
  [Q_rad_win5] -> Mux1/5
  From63/1 -> Subsystem4/2(In2)
  Discrete-Time Integrator1/1 -> MATLAB Function3/3(wallTempOuter)
  Demux1/11 -> [deltaTPartition11]
  [Q_rad_win11] -> Mux1/11
  [T_7] -> Mux/7
  [deltaTWalls] -> Discrete-Time Integrator1/1
  Product6/1 -> Display2/1, Goto33/1
  Demux1/6 -> [deltaTPartition6]
  Constant13/1 -> Discrete-Time Integrator1/2
  Demux1/10 -> [deltaTPartition10]
  [Q_rad_win1] -> Mux1/1
  [T_10] -> Mux/10
  [T_3] -> Mux/3
  Demux1/9 -> [deltaTPartition9]
  [Q_rad_win4] -> Mux1/4
  [T_11] -> Mux/11
  Demux1/4 -> [deltaTPartition4]
  Mux1/1 -> MATLAB Function3/2(irradianceToRoom)
  [T_1] -> Mux/1
  roomAirHeatCapcities/1 -> Product5/2
  From87/1 -> Subsystem4/3(In3)
  [T_6] -> Mux/6
  Demux1/3 -> [deltaTPartition3]
  Subsystem4/1(Out1) -> Product6/1
  [T_9] -> Mux/9

== system Final_Model_Building_2_AirflowAdded_BufferMode/ASHP_Subsystem ==
  DHW for ASHP Case : Subsystem
  Defrost Timer : Subsystem
  Delay : Delay  DelayLength=1  InitialCondition=0
  Delay1 : Delay  DelayLength=1  InitialCondition=0
  Delay2 : Delay  DelayLength=5  InitialCondition=0
  Discrete-Time Integrator : DiscreteIntegrator  ExternalReset=falling  SampleTime=-1  LimitOutput=on  UpperSaturationLimit=1  LowerSaturationLimit=0  ICPrevOutput=DiscIntNeverNeededParam  ICPrevScaledInput=DiscIntNeverNeededParam
  Divide : Product  Inputs=*/
  Fixed pump heating rate 1 l/s : Constant
  Heat sys act? : Constant
  Logical Operator : Logic  Operator=NOT  Inputs=1  AllPortsSameDT=off  OutDataTypeStr=boolean
  Saturation : Saturate  UpperLimit=1  LowerLimit=0
  Scope2 : Scope
  Subsystem14 : Subsystem  TreatAsAtomicUnit=on
      mask Display:
      | port_label('input', 1, 'T_Out')
      | port_label('input', 2, 'NormalOn')
      | port_label('input', 3, 'DefrostOn')
      | port_label('input', 4, 'MixedTemp')
      | port_label('input', 5, 'MassFlowTotal')
      | port_label('input', 6, 'GCS')
      | port_label('input', 7, 'SHSig')
      | 
      | 
      | port_label('output', 1, 'Hysteresis')
      | port_label('output', 2, 'THB_to_Pre')
      | port_label('output', 3, 'd_signal')
      | port_label('output', 4, 'n_signal')
      | port_label('output', 5, 'Therm_out')
      | port_label('output', 6, 'Elec_out')
      | 
      | disp('SH_ASHP')
  Sum1 : Sum
  Sum2 : Sum  Inputs=2
  Sum3 : Sum
  Sum4 : Sum
  Time in seconds for Heat pump to reach full stady state output : Constant  Value=pumpRamp
  Water Demand Time Series (Minute) : Constant  Value=DHWDemandProfile
  mains water temp : Constant  Value=12
  tag scope: AuxHeatToWater=global, DHW_heating_on=global, DefrostOn=global, ElectrifiedHeatToSpace=global, ElectrifiedHeatToWater=global, HeatPumpFlow=global, HeatToSpace=global, HeatToWater=global, NormalOn=global, SH_Signal=global, THB_In_Pre=global, d_signal=global, hysteresis=global, n_signal=global, pump_power_Fraction=global
  wires:
  [n_signal] -> Delay1/1
  Time in seconds for Heat pump to reach full stady state output/1 -> Divide/2
  Subsystem14/1(Out1) -> [hysteresis]
  Sum1/1 -> Sum4/1, [d_signal]
  Saturation/1 -> Defrost Timer/3(In3)
  [d_signal] -> Delay/1
  Sum4/1 -> Discrete-Time Integrator/2, Divide/1
  [T_Out] -> Subsystem14/1(In1)
  Subsystem14/5(Out5) -> [HeatToSpace]
  Discrete-Time Integrator/1 -> Delay2/1
  [SH_Signal] -> Subsystem14/7(In7)
  DHW for ASHP Case/5(Out5) -> [ElectrifiedHeatToWater]
  [T_Out] -> DHW for ASHP Case/2(In2)
  DHW for ASHP Case/6(Out6) -> [AuxHeatToWater]
  Delay2/1 -> [pump_power_Fraction]
  Subsystem14/2(Out2) -> [THB_In_Pre]
  [Pump_Return] -> Subsystem14/4(In4)
  [pump_power_Fraction] -> Subsystem14/8(In8)
  Subsystem14/4(Out4) -> Sum3/1
  Water Demand Time Series (Minute)/1 -> DHW for ASHP Case/5(In5)
  [Global_Control_Signal] -> Subsystem14/6(In6)
  Divide/1 -> Discrete-Time Integrator/1
  Subsystem14/6(Out6) -> [ElectrifiedHeatToSpace]
  [T_1] -> DHW for ASHP Case/1(In1)
  Heat sys act?/1 -> Defrost Timer/2(In2)
  Delay1/1 -> Sum2/2
  Delay/1 -> Sum2/1
  Fixed pump heating rate 1 l/s/1 -> Subsystem14/5(In5)
  Defrost Timer/2(Out2) -> [DefrostOn]
  DHW for ASHP Case/1(Out1) -> Scope2/1
  DHW for ASHP Case/7(Out7) -> [HeatToWater]
  DHW for ASHP Case/4(Out4) -> Sum3/2
  [DefrostOn] -> DHW for ASHP Case/4(In4)
  Subsystem14/3(Out3) -> Sum1/1
  DHW for ASHP Case/3(Out3) -> Sum1/2
  Sum3/1 -> Sum4/2, [n_signal]
  Defrost Timer/1(Out1) -> [NormalOn]
  Sum2/1 -> Saturation/1
  [DefrostOn] -> Subsystem14/3(In3)
  [T_Out] -> Defrost Timer/1(In1)
  [NormalOn] -> Subsystem14/2(In2)
  [NormalOn] -> DHW for ASHP Case/3(In3)
  DHW for ASHP Case/2(Out2) -> [DHW_heating_on]
  mains water temp/1 -> DHW for ASHP Case/6(In6)
  [DHW_heating_on] -> Logical Operator/1
  Logical Operator/1 -> [SH_Signal]
  Subsystem14/7(Out7) -> [HeatPumpFlow]

== system Final_Model_Building_2_AirflowAdded_BufferMode/ASHP_Subsystem_Variable ==
  DHW for ASHP Case : Subsystem
  Defrost Timer : Subsystem
  Delay : Delay  DelayLength=1  InitialCondition=0
  Delay1 : Delay  DelayLength=1  InitialCondition=0
  Delay2 : Delay  DelayLength=5  InitialCondition=0
  Discrete-Time Integrator : DiscreteIntegrator  ExternalReset=falling  SampleTime=-1  LimitOutput=on  UpperSaturationLimit=1  LowerSaturationLimit=0  ICPrevOutput=DiscIntNeverNeededParam  ICPrevScaledInput=DiscIntNeverNeededParam
  Divide : Product  Inputs=*/
  Fixed pump heating rate 1 l/s : Constant
  Heat sys act? : Constant
  Logical Operator : Logic  Operator=NOT  Inputs=1  AllPortsSameDT=off  OutDataTypeStr=boolean
  Saturation : Saturate  UpperLimit=1  LowerLimit=0
  Scope1 : Scope
  Scope16 : Scope  NumInputPorts=2
  Scope2 : Scope
  Scope3 : Scope
  Subsystem : Subsystem
      mask Display:
      | port_label('input', 1, 'T_outside')
      | port_label('input', 2, 'Normal_On')
      | port_label('input', 3, 'Defrost_On')
      | port_label('input', 4, 'returnTemp')
      | port_label('input', 5, 'm_dot_FullOn')
      | port_label('input', 6, 'GCS')
      | port_label('input', 7, 'SH')
      | 
      | port_label('output', 1, 'THB_to_Pre')
      | port_label('output', 2, 'Hysteresis')
      | port_label('output', 3, 'D_signal')
      | port_label('output', 4, 'N_signal')
      | port_label('output', 5, 'ElecOut')
      | port_label('output', 6, 'ThermOut')
  Sum1 : Sum
  Sum2 : Sum  Inputs=2
  Sum3 : Sum
  Sum4 : Sum
  Time in seconds for Heat pump to reach full stady state output : Constant  Value=pumpRamp
  Water Demand Time Series (Minute) : Constant  Value=DHWDemandProfile
  mains water temp : Constant  Value=12
  tag scope: AuxHeatToWater=global, DHW_heating_on=global, DefrostOn=global, ElectrifiedHeatToSpace=global, ElectrifiedHeatToWater=global, HeatPumpFlow=global, HeatToSpace=global, HeatToWater=global, NormalOn=global, SH_Signal=global, THB_In_Pre=global, d_signal=global, hysteresis=global, n_signal=global, pump_power_Fraction=global
  wires:
  [n_signal] -> Delay1/1
  Subsystem/2(Out2) -> [hysteresis]
  Sum1/1 -> Sum4/1, [d_signal]
  Saturation/1 -> Defrost Timer/3(In3)
  [d_signal] -> Delay/1
  [T_Out] -> Subsystem/1(In1)
  Subsystem/6(Out6) -> Scope16/1, [HeatToSpace]
  [SH_Signal] -> Subsystem/7(In7)
  DHW for ASHP Case/5(Out5) -> [ElectrifiedHeatToWater]
  [T_Out] -> DHW for ASHP Case/2(In2)
  DHW for ASHP Case/6(Out6) -> [AuxHeatToWater]
  Subsystem/1(Out1) -> Scope1/1, [THB_In_Pre]
  [Pump_Return] -> Subsystem/4(In4)
  Subsystem/4(Out4) -> Sum3/1
  Water Demand Time Series (Minute)/1 -> DHW for ASHP Case/5(In5)
  [Global_Control_Signal] -> Subsystem/6(In6)
  Subsystem/5(Out5) -> Scope16/2, [ElectrifiedHeatToSpace]
  [T_1] -> DHW for ASHP Case/1(In1)
  Heat sys act?/1 -> Defrost Timer/2(In2)
  Delay1/1 -> Sum2/2
  Delay/1 -> Sum2/1
  Defrost Timer/2(Out2) -> Scope3/1, [DefrostOn]
  DHW for ASHP Case/1(Out1) -> Scope2/1
  DHW for ASHP Case/7(Out7) -> [HeatToWater]
  DHW for ASHP Case/4(Out4) -> Sum3/2
  [DefrostOn] -> DHW for ASHP Case/4(In4)
  Subsystem/3(Out3) -> Sum1/1
  DHW for ASHP Case/3(Out3) -> Sum1/2
  Sum3/1 -> Sum4/2, [n_signal]
  Defrost Timer/1(Out1) -> [NormalOn]
  Sum2/1 -> Saturation/1
  [DefrostOn] -> Subsystem/3(In3)
  [T_Out] -> Defrost Timer/1(In1)
  [NormalOn] -> Subsystem/2(In2)
  [NormalOn] -> DHW for ASHP Case/3(In3)
  DHW for ASHP Case/2(Out2) -> [DHW_heating_on]
  mains water temp/1 -> DHW for ASHP Case/6(In6)
  [DHW_heating_on] -> Logical Operator/1
  Logical Operator/1 -> [SH_Signal]
  Discrete-Time Integrator/1 -> Delay2/1
  Sum4/1 -> Discrete-Time Integrator/2, Divide/1
  Delay2/1 -> [pump_power_Fraction]
  Time in seconds for Heat pump to reach full stady state output/1 -> Divide/2
  Divide/1 -> Discrete-Time Integrator/1
  [pump_power_Fraction] -> Subsystem/8(In8)
  Subsystem/7(Out7) -> [HeatPumpFlow]
  Fixed pump heating rate 1 l/s/1 -> Subsystem/5(In5)
